simulink model "mechanical_characteristic_prsAD"  (R2015b)
settings: Solver=ode4  StartTime=0.0  StopTime=inf  FixedStep=2e-5  MaxStep=1e-6  RelTol=1e-6
libraries: powerlib x33, powerlib_meascontrol x4, simulink x1
settings Model: ExtModeTrigDuration=100  Creator=Alexey  LastModifiedBy=Артем
settings SolverCC: MaxConsecutiveZCs=1000000  ZeroCrossControl=DisableAll
settings DataIOCC: Decimation=10  LimitDataPoints=off  SaveFinalState=on  SaveFormat=StructureWithTime  SignalLoggingSaveFormat=ModelDataLogs  SaveOutput=off  SaveState=on  StateSaveName=tmp_raccel_xout  SignalLoggingName=tmp_raccel_logsout
settings OptimizationCC: ExpressionDepthLimit=2147483647  InitFltsAndDblsToZero=on  EfficientMapNaN2IntZero=off
settings DebuggingCC: SaveWithParameterizedLinksMsg=none  UnderspecifiedInitializationDetection=Classic  MergeDetectMultiDrivingBlocksExec=none  SignalResolutionControl=TryResolveAllWithWarning  SolverPrmCheckMsg=warning  MultiTaskDSMMsg=warning  MultiTaskCondExecSysMsg=none  FcnCallInpInsideContextMsg=UseLocalSettings  UnconnectedInputMsg=none  UnconnectedOutputMsg=none  UnconnectedLineMsg=none  StateNameClashWarn=warning
settings HardwareCC: ProdBitPerPointer=32  ProdLargestAtomicFloat=None  ProdIntDivRoundTo=Undefined  ProdEndianess=Unspecified  ProdWordSize=32  ProdHWDeviceType=32-bit Generic  TargetBitPerPointer=64  TargetLongLongMode=on  TargetIntDivRoundTo=Zero  TargetEndianess=LittleEndian  TargetWordSize=64  TargetHWDeviceType=MATLAB Host  ProdEqTarget=off
settings RTWCC: SystemTargetFile=raccel.tlc  TemplateMakefile=raccel_default_tmf  RTWVerbose=off  RTWUseSimCustomCode=on
settings CodeAppCC: GenerateComments=off  MaxIdLength=128  MangleLength=10  SimulinkBlockComments=off
settings RaccelTargetCC: ERTMultiwordTypeDef=System defined  ERTMultiwordLength=256  GeneratePreprocessorConditionals=Use local settings  ERTFirstTimeCompliant=off  MultiInstanceERTCode=off  ENABLE_SLEXEC_SSBRIDGE=0  RTWCAPIParams=on
settings ConfigComp: CovModelRefEnable=Off

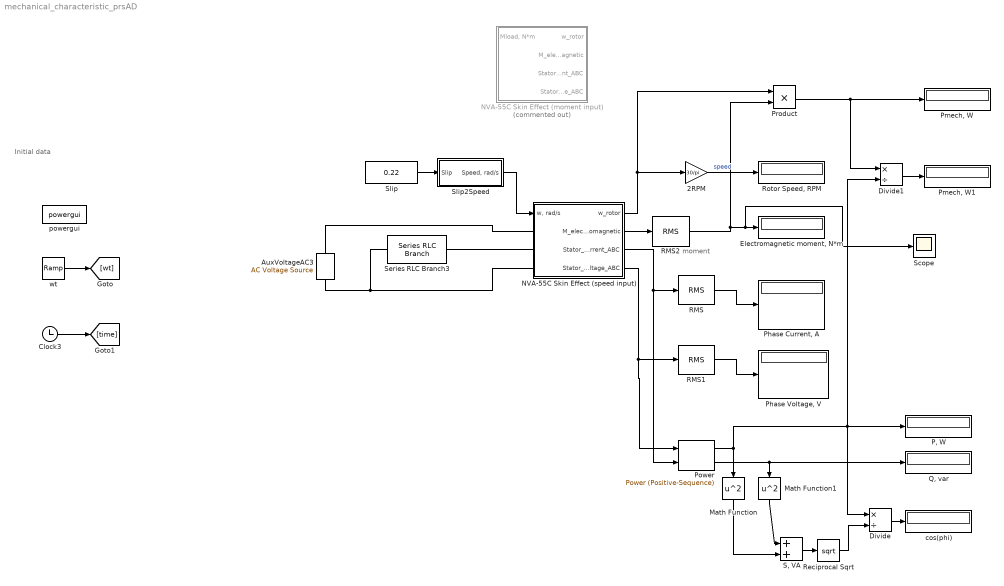
== system mechanical_characteristic_prsAD ==
  note: Initial data
  note: moment
  2RPM : Gain  Gain=30/pi
  AuxVoltageAC3 : powerlib/Electrical Sources/AC Voltage Source  Amplitude=278*sqrt(2)  Phase=0  Frequency=50  SampleTime=0  Measurements=None  BusType=swing  Pref=10e3  Qref=0  Qmin=-inf  Qmax=+inf
  Clock3 : Clock
  Divide : Product  Inputs=*/
  Divide1 : Product  Inputs=*/
  "Electromagnetic moment, N*m" : Display
  Math Function : Math  Operator=square  SaturateOnIntegerOverflow=on
  Math Function1 : Math  Operator=square  SaturateOnIntegerOverflow=on
  NVA-55C Skin Effect (moment input) : Subsystem  RequirementInfo={} %GIDa_83907570_a8f5_4683_9026_05a41bdf487c  Commented=on  mask(Модель асинхронной машины){f_nominal=50, Rs=0.0472, ls=0.0003883, Rr=0.0392, lr=0.0005399, Lm=0.011, Zp=2, Jr=1.25, l_s=326, q_s=119.52, n_2=38, d_r=207.4, q_r=498.1, h_p=3}
      mask prompts: f_nominal "Номинальная частота, Гц"; Rs "Активное сопротивление статора, Ом"; ls "Индуктивность статора, Гн"; Rr "Активное сопротивление ротора, Ом"; lr "Индуктивность ротора, Гн"; Lm "Взаимная индуктивность, Гн"; Zp "Число пар полюсов"; Jr "Коэффициент инерции ротора, кг*м^2"; l_s "Длина стержня ротора, мм"; q_s "Площадь поперечного сечения стержня, мм^2"; n_2 "Число пазов ротора"; d_r "Средний диаметр кольца, мм"; q_r "Площадь поперечного сечения кольца, мм^2"; h_p "Глубина паза, см"
      mask help: Описание
      mask init:
      | Ls = ls + Lm;
      | Lr = lr + Lm;
      | Kr = Lm / Lr;
      | Ks = Lm / Ls;
      | sigma = 1 - (Lm ^ 2) / (Ls * Lr);
      | 
      | dol_paz = (l_s / q_s) / ((l_s / q_s) + (n_2 * d_r) / (q_r * 2 * pi * Zp ^ 2));
      | dol_lob = ((n_2 * d_r) / (q_r * 2 * pi * Zp ^ 2))/ ((l_s / q_s) + (n_2 * d_r) / (q_r * 2 * pi * Zp ^ 2));
      | 
      | w_s = (2 * pi * f_nominal) / Zp;
  NVA-55C Skin Effect (speed input) : Subsystem  RequirementInfo={} %GIDa_29323b18_8ff0_47b3_9951_5813d07141ee  mask(Модель асинхронной машины){f_nominal=50, Rs=0.0472, ls=0.0003883, Rr=0.0392, lr=0.0005399, Lm=0.011, Zp=2, Jr=1.25, l_s=326, q_s=119.52, n_2=38, d_r=207.4, q_r=498.1, h_p=3}
      mask prompts: f_nominal "Номинальная частота, Гц"; Rs "Активное сопротивление статора, Ом"; ls "Индуктивность статора, Гн"; Rr "Активное сопротивление ротора, Ом"; lr "Индуктивность ротора, Гн"; Lm "Взаимная индуктивность, Гн"; Zp "Число пар полюсов"; Jr "Коэффициент инерции ротора, кг*м^2"; l_s "Длина стержня ротора, мм"; q_s "Площадь поперечного сечения стержня, мм^2"; n_2 "Число пазов ротора"; d_r "Средний диаметр кольца, мм"; q_r "Площадь поперечного сечения кольца, мм^2"; h_p "Глубина паза, см"
      mask help: Описание
      mask init: same as mechanical_characteristic_prsAD/NVA-55C Skin Effect (moment input)
  "P, W" : Display
  "Phase Current, A" : Display
  "Phase Voltage, V" : Display
  "Pmech, W" : Display
  "Pmech, W1" : Display
  Power : powerlib_meascontrol/Measurements/Power (Positive-Sequence)  Freq=50  Vinit=[0, 0]  Iinit=[0, 0]  Ts=0
  Product : Product
  "Q, var" : Display
  RMS : powerlib_meascontrol/Measurements/RMS  TrueRMS=on  Freq=50  RMSInit=0  Ts=0
  RMS1 : powerlib_meascontrol/Measurements/RMS  TrueRMS=on  Freq=50  RMSInit=0  Ts=0
  RMS2 : powerlib_meascontrol/Measurements/RMS  TrueRMS=on  Freq=50  RMSInit=0  Ts=0
  Reciprocal Sqrt : Sqrt  SaturateOnIntegerOverflow=on
  "Rotor Speed, RPM" : Display
  "S, VA" : Sum
  Scope : Scope
  Series RLC Branch3 : powerlib/Elements/Series RLC Branch  LConnTagsString=__new0  RConnTagsString=__new0  BranchType=C  Resistance=0  Inductance=0  SetiL0=off  InitialCurrent=0  Capacitance=2160e-6  Setx0=off  InitialVoltage=0  Measurements=None
  Slip : Constant  Value=0.22
  Slip2Speed : Subsystem  mask(Slip2Speed){w1=1500}
      mask prompts: w1 "Синхронная частота вращения, об/мин"
  cos(phi) : Display
  powergui : powerlib/powergui  SimulationMode=Discrete  SolverType=Tustin  SampleTime=2e-5  frequency=50  SPID=off  DisableSnubberDevices=off  DisableRonSwitches=off  DisableVfSwitches=off  SwTol=0  DisplayEquations=off  Interpol=off  ExternalGateDelay=off  methode=off  Ts=0  FunctionMessages=off  echomessages=off  HookPort=off  EnableUseOfTLC=off  x0status=blocks  frequencyindice=50  Pbase=100e6  ErrMax=1e-4  Iterations=50  UnitsV=kV  UnitsW=MW  buscounter=0  RestoreLinks=warning  ResistiveCurrentMeasurement=off  Frange=[0:2:500]  Ylog=off  Xlog=on  ShowGrid=off  save=off  variable=ZData  structure=0  ZoomFFT=on  StartTime=0.0  cycles=1  DisplayStyle=1  fundamental=60  FreqAxis=off  MaxFrequency=1000  frequencyindicesteady=1  RmsSteady=1  display=off
  wt : simulink/Sources/Ramp  slope=2*pi*50  start=0  X0=0
  wires:
  wt/1 -> [wt]
  Clock3/1 -> [time]
  2RPM/1 -> "Rotor Speed, RPM"/1  "speed"
  Slip/1 -> Slip2Speed/1(Slip)
  Slip2Speed/1("Speed, rad/s") -> NVA-55C Skin Effect (speed input)/1("w, rad/s")
  NVA-55C Skin Effect (speed input)/2(M_electromagnetic) -> RMS2/1
  NVA-55C Skin Effect (speed input)/1(w_rotor) -> 2RPM/1, Product/1
  NVA-55C Skin Effect (speed input)/3(Stator_current_ABC) -> RMS/1, Power/2
  NVA-55C Skin Effect (speed input)/4(Stator_voltage_ABC) -> Power/1, RMS1/1
  RMS/1 -> "Phase Current, A"/1
  RMS1/1 -> "Phase Voltage, V"/1
  Power/1 -> Divide/1, "P, W"/1, Divide1/2, Math Function/1
  Power/2 -> "Q, var"/1, Math Function1/1
  "S, VA"/1 -> Reciprocal Sqrt/1
  Divide/1 -> cos(phi)/1
  Product/1 -> Divide1/1, "Pmech, W"/1
  Divide1/1 -> "Pmech, W1"/1
  Math Function/1 -> "S, VA"/2
  Math Function1/1 -> "S, VA"/1
  Reciprocal Sqrt/1 -> Divide/2
  RMS2/1 -> Product/2, Scope/1, "Electromagnetic moment, N*m"/1
  connections:
  Series RLC Branch3/RConn1 -- NVA-55C Skin Effect (speed input)/LConn2
  AuxVoltageAC3/LConn1 -- NVA-55C Skin Effect (speed input)/LConn3 -- Series RLC Branch3/LConn1
  AuxVoltageAC3/RConn1 -- NVA-55C Skin Effect (speed input)/LConn1

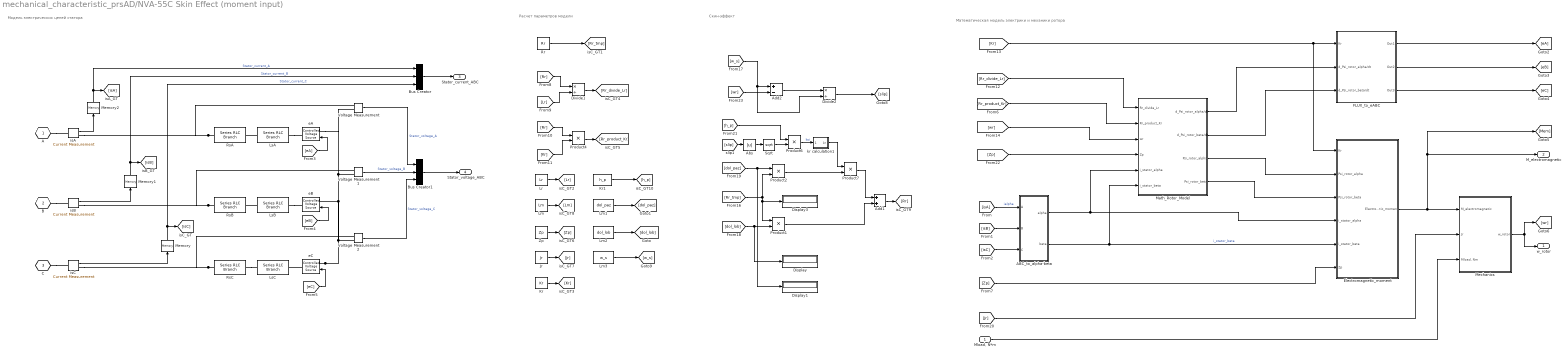
== system mechanical_characteristic_prsAD/NVA-55C Skin Effect (moment input) ==
  note: Модель электрических цепей статора
  note: Расчет параметров модели
  note: Математическая модель электрики и механики ротора
  note: Скин-эффект
  "Mload, N*m " : Inport
  ABC_to_alpha-beta : Subsystem
  Abs : Abs
  Add1 : Sum
  Add2 : Sum  Inputs=+-
  Bus Creator : BusCreator  Inputs=3
  Bus Creator1 : BusCreator  Inputs=3
  Display : Display
  Display1 : Display
  Display3 : Display
  Divide1 : Product  Inputs=*/
  Divide2 : Product  Inputs=*/
  "Electromagnetic_moment " : Subsystem
  FLUX_to_eABC : Subsystem
  Jr : Constant  Value=Jr
  Kr : Constant  Value=Kr
  Kr1 : Constant  Value=h_p
  Lm : Constant  Value=Lm
  Lm1 : Constant  Value=dol_paz
  Lm2 : Constant  Value=dol_lob
  Lm3 : Constant  Value=w_s
  Lr : Constant  Value=Lr
  LsA : powerlib/Elements/Series RLC Branch  LConnTagsString=__new0  RConnTagsString=__new0  BranchType=L  Resistance=Rs  Inductance=Ls * sigma  SetiL0=off  InitialCurrent=0  Capacitance=1e-6  Setx0=off  InitialVoltage=0  Measurements=None
  LsB : powerlib/Elements/Series RLC Branch  LConnTagsString=__new0  RConnTagsString=__new0  BranchType=L  Resistance=Rs  Inductance=Ls * sigma  SetiL0=off  InitialCurrent=0  Capacitance=1e-6  Setx0=off  InitialVoltage=0  Measurements=None
  LsC : powerlib/Elements/Series RLC Branch  LConnTagsString=__new0  RConnTagsString=__new0  BranchType=L  Resistance=Rs  Inductance=Ls * sigma  SetiL0=off  InitialCurrent=0  Capacitance=1e-6  Setx0=off  InitialVoltage=0  Measurements=None
  Math_Rotor_Model : Subsystem
  Mechanics : Subsystem
  Memory : Memory
  Memory1 : Memory
  Memory2 : Memory
  Product{1..2,4,6..7} (5 alike) : Product
  Rr : Constant  Value=Rr
  RsA : powerlib/Elements/Series RLC Branch  LConnTagsString=__new0  RConnTagsString=__new0  BranchType=R  Resistance=Rs  Inductance=1e-3  SetiL0=off  InitialCurrent=0  Capacitance=1e-6  Setx0=off  InitialVoltage=0  Measurements=None
  RsB : powerlib/Elements/Series RLC Branch  LConnTagsString=__new0  RConnTagsString=__new0  BranchType=R  Resistance=Rs  Inductance=1e-3  SetiL0=off  InitialCurrent=0  Capacitance=1e-6  Setx0=off  InitialVoltage=0  Measurements=None
  RsC : powerlib/Elements/Series RLC Branch  LConnTagsString=__new0  RConnTagsString=__new0  BranchType=R  Resistance=Rs  Inductance=1e-3  SetiL0=off  InitialCurrent=0  Capacitance=1e-6  Setx0=off  InitialVoltage=0  Measurements=None
  Sqrt : Sqrt  SaturateOnIntegerOverflow=on
  Voltage Measurement : powerlib/Measurements/Voltage Measurement  PhasorSimulation=off  OutputType=Complex  PSBequivalent=0
  Voltage Measurement1 : powerlib/Measurements/Voltage Measurement  PhasorSimulation=off  OutputType=Complex  PSBequivalent=0
  Voltage Measurement2 : powerlib/Measurements/Voltage Measurement  PhasorSimulation=off  OutputType=Complex  PSBequivalent=0
  Zp : Constant  Value=Zp
  eA : powerlib/Electrical Sources/Controlled Voltage Source  Initialize=on  Source_Type=AC  Amplitude=0  Phase=0  Frequency=0  Measurements=None
  eB : powerlib/Electrical Sources/Controlled Voltage Source  Initialize=on  Source_Type=AC  Amplitude=0  Phase=0  Frequency=0  Measurements=None
  eC : powerlib/Electrical Sources/Controlled Voltage Source  Initialize=on  Source_Type=AC  Amplitude=0  Phase=0  Frequency=0  Measurements=None
  isA : powerlib/Measurements/Current Measurement  PhasorSimulation=off  OutputType=Complex  PSBequivalent=0
  isB : powerlib/Measurements/Current Measurement  PhasorSimulation=off  OutputType=Complex  PSBequivalent=0
  isC : powerlib/Measurements/Current Measurement  PhasorSimulation=off  OutputType=Complex  PSBequivalent=0
  kr calculation1 : Subsystem
  A : PMIOPort  Tag=PMCPort  Port=1  Side=Left
  B : PMIOPort  Tag=PMCPort  Port=2  Side=Left
  C : PMIOPort  Tag=PMCPort  Port=3  Side=Left
  w_rotor : Outport
  M_electromagnetic : Outport  Port=2
  Stator_current_ABC : Outport  Port=3
  Stator_voltage_ABC : Outport  Port=4
  wires:
  kr calculation1/1(kr) -> Product7/1
  Bus Creator1/1 -> Stator_voltage_ABC/1
  Voltage Measurement2/1 -> Bus Creator1/3  "Stator_voltage_C"
  Voltage Measurement1/1 -> Bus Creator1/2  "Stator_voltage_B"
  Voltage Measurement/1 -> Bus Creator1/1  "Stator_voltage_A"
  Abs/1 -> Sqrt/1
  [slip] -> Abs/1
  [Jr] -> Mechanics/2(Jr)
  Divide2/1 -> [slip]
  Add2/1 -> Divide2/1
  [wr] -> Add2/2
  [w_s] -> Divide2/2, Add2/1
  Lm3/1 -> [w_s]
  Lm1/1 -> [dol_paz]
  Lm2/1 -> [dol_lob]
  Product7/1 -> Add1/1
  Product6/1 -> kr calculation1/1(ksi)  "ksi"
  Product2/1 -> Product7/2
  [h_p] -> Product6/1
  Sqrt/1 -> Product6/2
  Kr1/1 -> [h_p]
  Add1/1 -> [Rr]
  Product1/1 -> Add1/2
  [dol_paz] -> Product2/1, Display1/1
  [dol_lob] -> Product1/2, Display/1
  [Rr_tmp] -> Product2/2, Product1/1, Display3/1
  Rr/1 -> [Rr_tmp]
  [Zp] -> Math_Rotor_Model/4(Zp)
  [wr] -> Math_Rotor_Model/3(wr)
  [Zp] -> "Electromagnetic_moment "/6(Zp)
  Math_Rotor_Model/3(Psi_rotor_alpha) -> "Electromagnetic_moment "/2(Psi_rotor_alpha)
  Math_Rotor_Model/4(Psi_rotor_beta) -> "Electromagnetic_moment "/3(Psi_rotor_beta)
  Math_Rotor_Model/2(d_Psi_rotor_beta/dt) -> FLUX_to_eABC/3(d_Psi_rotor_beta/dt)
  Math_Rotor_Model/1(d_Psi_rotor_alpha/dt) -> FLUX_to_eABC/2(d_Psi_rotor_alpha/dt)
  [Rr_product_Kr] -> Math_Rotor_Model/2(Rr_product_Kr)
  [Rr_divide_Lr] -> Math_Rotor_Model/1(Rr_divide_Lr)
  FLUX_to_eABC/3(Out3) -> [eC]
  FLUX_to_eABC/2(Out2) -> [eB]
  FLUX_to_eABC/1(Out1) -> [eA]
  [Kr] -> FLUX_to_eABC/1(Kr), "Electromagnetic_moment "/1(Kr)
  "Electromagnetic_moment "/1(Electromagnetic_moment) -> [Mem], M_electromagnetic/1, Mechanics/1(M_electromagnetic)
  Bus Creator/1 -> Stator_current_ABC/1
  ABC_to_alpha-beta/1(alpha) -> "Electromagnetic_moment "/4(i_stator_alpha), Math_Rotor_Model/5(i_stator_alpha)
  [isC] -> ABC_to_alpha-beta/3(C)
  [isB] -> ABC_to_alpha-beta/2(B)
  ABC_to_alpha-beta/2(beta) -> "Electromagnetic_moment "/5(i_stator_beta), Math_Rotor_Model/6(i_stator_beta)  "i_stator_beta"
  Memory2/1 -> [isA], Bus Creator/1  "Stator_current_A"
  Memory1/1 -> [isB], Bus Creator/2  "Stator_current_B"
  Memory/1 -> [isC], Bus Creator/3  "Stator_current_C"
  isA/1 -> Memory2/1
  isB/1 -> Memory1/1
  isC/1 -> Memory/1
  Kr/1 -> [Kr]
  Lm/1 -> [Lm]
  [isA] -> ABC_to_alpha-beta/1(A)  "ialpha"
  Product4/1 -> [Rr_product_Kr]
  [Kr] -> Product4/2
  [Rr] -> Product4/1
  [eC] -> eC/1
  [eA] -> eA/1
  [eB] -> eB/1
  [Rr] -> Divide1/1
  Lr/1 -> [Lr]
  Jr/1 -> [Jr]
  Zp/1 -> [Zp]
  Divide1/1 -> [Rr_divide_Lr]
  [Lr] -> Divide1/2
  Mechanics/1(w_rotor) -> [wr], w_rotor/1
  "Mload, N*m "/1 -> Mechanics/3("Mload, Nm")
  connections:
  LsB/RConn1 -- eB/RConn1
  eC/LConn1 -- Voltage Measurement2/LConn2 -- eB/LConn1 -- Voltage Measurement1/LConn2 -- Voltage Measurement/LConn2 -- eA/LConn1
  LsA/RConn1 -- eA/RConn1
  eC/RConn1 -- LsC/RConn1
  RsA/LConn1 -- Voltage Measurement/LConn1 -- isA/RConn1
  A/RConn1 -- isA/LConn1
  RsB/LConn1 -- Voltage Measurement1/LConn1 -- isB/RConn1
  B/RConn1 -- isB/LConn1
  RsC/LConn1 -- Voltage Measurement2/LConn1 -- isC/RConn1
  C/RConn1 -- isC/LConn1
  LsA/LConn1 -- RsA/RConn1
  RsC/RConn1 -- LsC/LConn1
  LsB/LConn1 -- RsB/RConn1

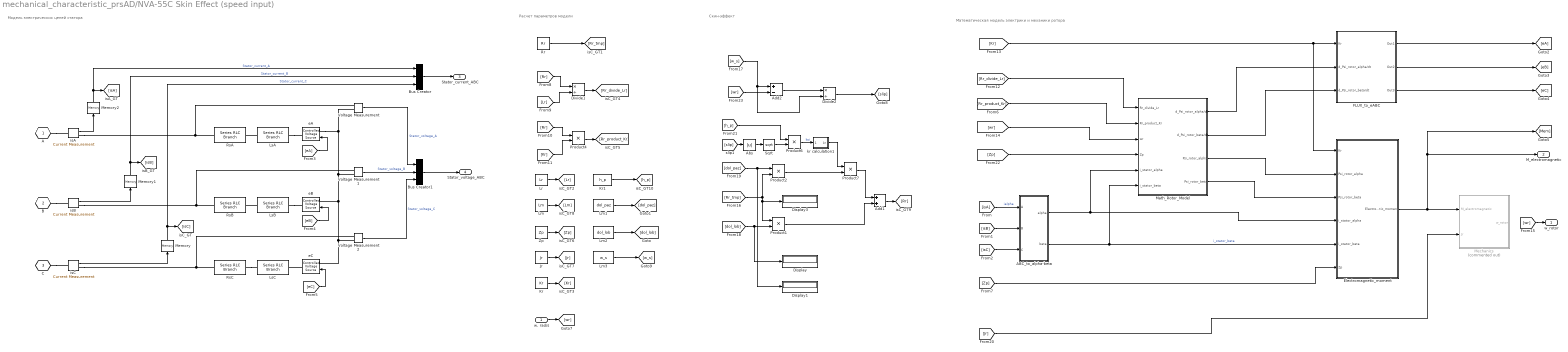
== system mechanical_characteristic_prsAD/NVA-55C Skin Effect (speed input) ==
  note: Скин-эффект
  note: Математическая модель электрики и механики ротора
  note: Расчет параметров модели
  note: Модель электрических цепей статора
  "w, rad/s" : Inport
  ABC_to_alpha-beta : Subsystem
  Abs : Abs
  Add1 : Sum
  Add2 : Sum  Inputs=+-
  Bus Creator : BusCreator  Inputs=3
  Bus Creator1 : BusCreator  Inputs=3
  Display : Display
  Display1 : Display
  Display3 : Display
  Divide1 : Product  Inputs=*/
  Divide2 : Product  Inputs=*/
  "Electromagnetic_moment " : Subsystem
  FLUX_to_eABC : Subsystem
  Jr : Constant  Value=Jr
  Kr : Constant  Value=Kr
  Kr1 : Constant  Value=h_p
  Lm : Constant  Value=Lm
  Lm1 : Constant  Value=dol_paz
  Lm2 : Constant  Value=dol_lob
  Lm3 : Constant  Value=w_s
  Lr : Constant  Value=Lr
  LsA : powerlib/Elements/Series RLC Branch  LConnTagsString=__new0  RConnTagsString=__new0  BranchType=L  Resistance=Rs  Inductance=Ls * sigma  SetiL0=off  InitialCurrent=0  Capacitance=1e-6  Setx0=off  InitialVoltage=0  Measurements=None
  LsB : powerlib/Elements/Series RLC Branch  LConnTagsString=__new0  RConnTagsString=__new0  BranchType=L  Resistance=Rs  Inductance=Ls * sigma  SetiL0=off  InitialCurrent=0  Capacitance=1e-6  Setx0=off  InitialVoltage=0  Measurements=None
  LsC : powerlib/Elements/Series RLC Branch  LConnTagsString=__new0  RConnTagsString=__new0  BranchType=L  Resistance=Rs  Inductance=Ls * sigma  SetiL0=off  InitialCurrent=0  Capacitance=1e-6  Setx0=off  InitialVoltage=0  Measurements=None
  Math_Rotor_Model : Subsystem
  Mechanics : Subsystem  Commented=on
  Memory : Memory
  Memory1 : Memory
  Memory2 : Memory
  Product{1..2,4,6..7} (5 alike) : Product
  Rr : Constant  Value=Rr
  RsA : powerlib/Elements/Series RLC Branch  LConnTagsString=__new0  RConnTagsString=__new0  BranchType=R  Resistance=Rs  Inductance=1e-3  SetiL0=off  InitialCurrent=0  Capacitance=1e-6  Setx0=off  InitialVoltage=0  Measurements=None
  RsB : powerlib/Elements/Series RLC Branch  LConnTagsString=__new0  RConnTagsString=__new0  BranchType=R  Resistance=Rs  Inductance=1e-3  SetiL0=off  InitialCurrent=0  Capacitance=1e-6  Setx0=off  InitialVoltage=0  Measurements=None
  RsC : powerlib/Elements/Series RLC Branch  LConnTagsString=__new0  RConnTagsString=__new0  BranchType=R  Resistance=Rs  Inductance=1e-3  SetiL0=off  InitialCurrent=0  Capacitance=1e-6  Setx0=off  InitialVoltage=0  Measurements=None
  Sqrt : Sqrt  SaturateOnIntegerOverflow=on
  Voltage Measurement : powerlib/Measurements/Voltage Measurement  PhasorSimulation=off  OutputType=Complex  PSBequivalent=0
  Voltage Measurement1 : powerlib/Measurements/Voltage Measurement  PhasorSimulation=off  OutputType=Complex  PSBequivalent=0
  Voltage Measurement2 : powerlib/Measurements/Voltage Measurement  PhasorSimulation=off  OutputType=Complex  PSBequivalent=0
  Zp : Constant  Value=Zp
  eA : powerlib/Electrical Sources/Controlled Voltage Source  Initialize=on  Source_Type=AC  Amplitude=0  Phase=0  Frequency=0  Measurements=None
  eB : powerlib/Electrical Sources/Controlled Voltage Source  Initialize=on  Source_Type=AC  Amplitude=0  Phase=0  Frequency=0  Measurements=None
  eC : powerlib/Electrical Sources/Controlled Voltage Source  Initialize=on  Source_Type=AC  Amplitude=0  Phase=0  Frequency=0  Measurements=None
  isA : powerlib/Measurements/Current Measurement  PhasorSimulation=off  OutputType=Complex  PSBequivalent=0
  isB : powerlib/Measurements/Current Measurement  PhasorSimulation=off  OutputType=Complex  PSBequivalent=0
  isC : powerlib/Measurements/Current Measurement  PhasorSimulation=off  OutputType=Complex  PSBequivalent=0
  kr calculation1 : Subsystem
  A : PMIOPort  Tag=PMCPort  Port=1  Side=Left
  B : PMIOPort  Tag=PMCPort  Port=2  Side=Left
  C : PMIOPort  Tag=PMCPort  Port=3  Side=Left
  w_rotor : Outport
  M_electromagnetic : Outport  Port=2
  Stator_current_ABC : Outport  Port=3
  Stator_voltage_ABC : Outport  Port=4
  wires:
  [wr] -> w_rotor/1
  "w, rad/s"/1 -> [wr]
  [Lr] -> Divide1/2
  Divide1/1 -> [Rr_divide_Lr]
  Zp/1 -> [Zp]
  Jr/1 -> [Jr]
  Lr/1 -> [Lr]
  [Rr] -> Divide1/1
  [eB] -> eB/1
  [eA] -> eA/1
  [eC] -> eC/1
  [Rr] -> Product4/1
  [Kr] -> Product4/2
  Product4/1 -> [Rr_product_Kr]
  [isA] -> ABC_to_alpha-beta/1(A)  "ialpha"
  Lm/1 -> [Lm]
  Kr/1 -> [Kr]
  isC/1 -> Memory/1
  isB/1 -> Memory1/1
  isA/1 -> Memory2/1
  Memory/1 -> Bus Creator/3, [isC]  "Stator_current_C"
  Memory1/1 -> Bus Creator/2, [isB]  "Stator_current_B"
  Memory2/1 -> Bus Creator/1, [isA]  "Stator_current_A"
  ABC_to_alpha-beta/2(beta) -> Math_Rotor_Model/6(i_stator_beta), "Electromagnetic_moment "/5(i_stator_beta)  "i_stator_beta"
  [isB] -> ABC_to_alpha-beta/2(B)
  [isC] -> ABC_to_alpha-beta/3(C)
  ABC_to_alpha-beta/1(alpha) -> Math_Rotor_Model/5(i_stator_alpha), "Electromagnetic_moment "/4(i_stator_alpha)
  Bus Creator/1 -> Stator_current_ABC/1
  "Electromagnetic_moment "/1(Electromagnetic_moment) -> Mechanics/1(M_electromagnetic), M_electromagnetic/1, [Mem]
  [Kr] -> "Electromagnetic_moment "/1(Kr), FLUX_to_eABC/1(Kr)
  FLUX_to_eABC/1(Out1) -> [eA]
  FLUX_to_eABC/2(Out2) -> [eB]
  FLUX_to_eABC/3(Out3) -> [eC]
  [Rr_divide_Lr] -> Math_Rotor_Model/1(Rr_divide_Lr)
  [Rr_product_Kr] -> Math_Rotor_Model/2(Rr_product_Kr)
  Math_Rotor_Model/1(d_Psi_rotor_alpha/dt) -> FLUX_to_eABC/2(d_Psi_rotor_alpha/dt)
  Math_Rotor_Model/2(d_Psi_rotor_beta/dt) -> FLUX_to_eABC/3(d_Psi_rotor_beta/dt)
  Math_Rotor_Model/4(Psi_rotor_beta) -> "Electromagnetic_moment "/3(Psi_rotor_beta)
  Math_Rotor_Model/3(Psi_rotor_alpha) -> "Electromagnetic_moment "/2(Psi_rotor_alpha)
  [Zp] -> "Electromagnetic_moment "/6(Zp)
  [wr] -> Math_Rotor_Model/3(wr)
  [Zp] -> Math_Rotor_Model/4(Zp)
  Rr/1 -> [Rr_tmp]
  [Rr_tmp] -> Display3/1, Product1/1, Product2/2
  [dol_lob] -> Display/1, Product1/2
  [dol_paz] -> Display1/1, Product2/1
  Product1/1 -> Add1/2
  Add1/1 -> [Rr]
  Kr1/1 -> [h_p]
  Sqrt/1 -> Product6/2
  [h_p] -> Product6/1
  Product2/1 -> Product7/2
  Product6/1 -> kr calculation1/1(ksi)  "ksi"
  Product7/1 -> Add1/1
  Lm2/1 -> [dol_lob]
  Lm1/1 -> [dol_paz]
  Lm3/1 -> [w_s]
  [w_s] -> Add2/1, Divide2/2
  [wr] -> Add2/2
  Add2/1 -> Divide2/1
  Divide2/1 -> [slip]
  [Jr] -> Mechanics/2(Jr)
  [slip] -> Abs/1
  Abs/1 -> Sqrt/1
  Voltage Measurement/1 -> Bus Creator1/1  "Stator_voltage_A"
  Voltage Measurement1/1 -> Bus Creator1/2  "Stator_voltage_B"
  Voltage Measurement2/1 -> Bus Creator1/3  "Stator_voltage_C"
  Bus Creator1/1 -> Stator_voltage_ABC/1
  kr calculation1/1(kr) -> Product7/1
  connections:
  LsB/LConn1 -- RsB/RConn1
  RsC/RConn1 -- LsC/LConn1
  LsA/LConn1 -- RsA/RConn1
  C/RConn1 -- isC/LConn1
  isC/RConn1 -- Voltage Measurement2/LConn1 -- RsC/LConn1
  B/RConn1 -- isB/LConn1
  isB/RConn1 -- Voltage Measurement1/LConn1 -- RsB/LConn1
  A/RConn1 -- isA/LConn1
  isA/RConn1 -- Voltage Measurement/LConn1 -- RsA/LConn1
  eC/RConn1 -- LsC/RConn1
  LsA/RConn1 -- eA/RConn1
  eA/LConn1 -- Voltage Measurement/LConn2 -- Voltage Measurement1/LConn2 -- eB/LConn1 -- Voltage Measurement2/LConn2 -- eC/LConn1
  LsB/RConn1 -- eB/RConn1

== system mechanical_characteristic_prsAD/Slip2Speed ==
  Slip : Inport
  Divide : Product  Inputs=**
  Subtract : Sum  Inputs=+-
  one1 : Constant
  one2 : Constant  Value=w1
  to rad/s : Gain  Gain=pi/30
  "Speed, rad/s" : Outport
  wires:
  Subtract/1 -> Divide/1
  one1/1 -> Subtract/1
  Divide/1 -> to rad/s/1
  to rad/s/1 -> "Speed, rad/s"/1
  Slip/1 -> Subtract/2
  one2/1 -> Divide/2

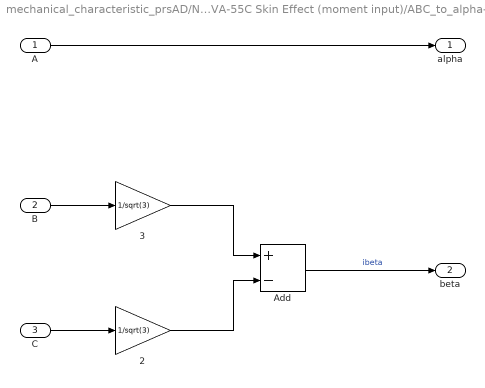
== system mechanical_characteristic_prsAD/NVA-55C Skin Effect (moment input)/ABC_to_alpha-beta ==
  A : Inport
  B : Inport  Port=2
  C : Inport  Port=3
  2 : Gain  Gain=1/sqrt(3)
  3 : Gain  Gain=1/sqrt(3)
  Add : Sum  Inputs=+-
  alpha : Outport
  beta : Outport  Port=2
  wires:
  A/1 -> alpha/1
  2/1 -> Add/2
  Add/1 -> beta/1  "ibeta"
  C/1 -> 2/1
  B/1 -> 3/1
  3/1 -> Add/1

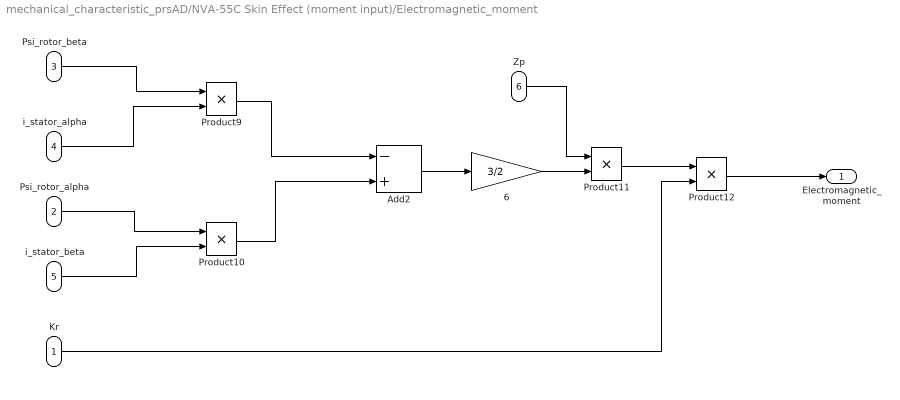
== system mechanical_characteristic_prsAD/NVA-55C Skin Effect (moment input)/Electromagnetic_moment  ==
  Kr : Inport
  Psi_rotor_alpha : Inport  Port=2
  Psi_rotor_beta : Inport  Port=3
  i_stator_alpha : Inport  Port=4
  i_stator_beta : Inport  Port=5
  Zp : Inport  Port=6
  6 : Gain  Gain=3/2
  Add2 : Sum  Inputs=-+
  Product{9..12} (4 alike) : Product
  Electromagnetic_moment : Outport
  wires:
  i_stator_beta/1 -> Product10/2
  Psi_rotor_beta/1 -> Product9/1
  Psi_rotor_alpha/1 -> Product10/1
  i_stator_alpha/1 -> Product9/2
  Add2/1 -> 6/1
  Zp/1 -> Product11/1
  6/1 -> Product11/2
  Product12/1 -> Electromagnetic_moment/1
  Product9/1 -> Add2/1
  Product10/1 -> Add2/2
  Kr/1 -> Product12/2
  Product11/1 -> Product12/1

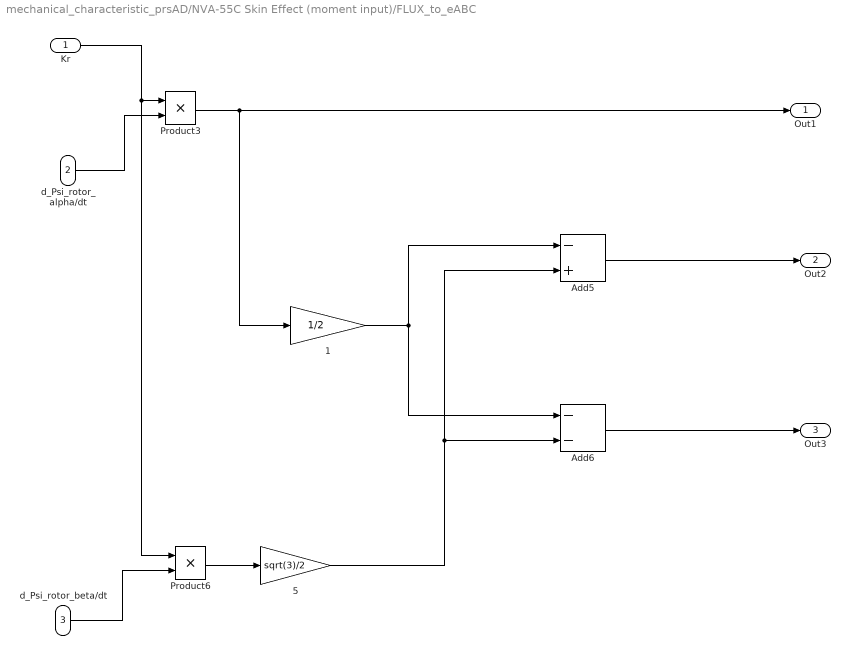
== system mechanical_characteristic_prsAD/NVA-55C Skin Effect (moment input)/FLUX_to_eABC ==
  Kr : Inport
  d_Psi_rotor_alpha/dt : Inport  Port=2
  d_Psi_rotor_beta/dt : Inport  Port=3
  1 : Gain  Gain=1/2
  5 : Gain  Gain=sqrt(3)/2
  Add5 : Sum  Inputs=-+
  Add6 : Sum  Inputs=--
  Product3 : Product
  Product6 : Product
  Out1 : Outport
  Out2 : Outport  Port=2
  Out3 : Outport  Port=3
  wires:
  d_Psi_rotor_beta/dt/1 -> Product6/2
  d_Psi_rotor_alpha/dt/1 -> Product3/2
  Add5/1 -> Out2/1
  Product3/1 -> 1/1, Out1/1
  Kr/1 -> Product3/1, Product6/1
  Add6/1 -> Out3/1
  5/1 -> Add6/2, Add5/2
  1/1 -> Add6/1, Add5/1
  Product6/1 -> 5/1

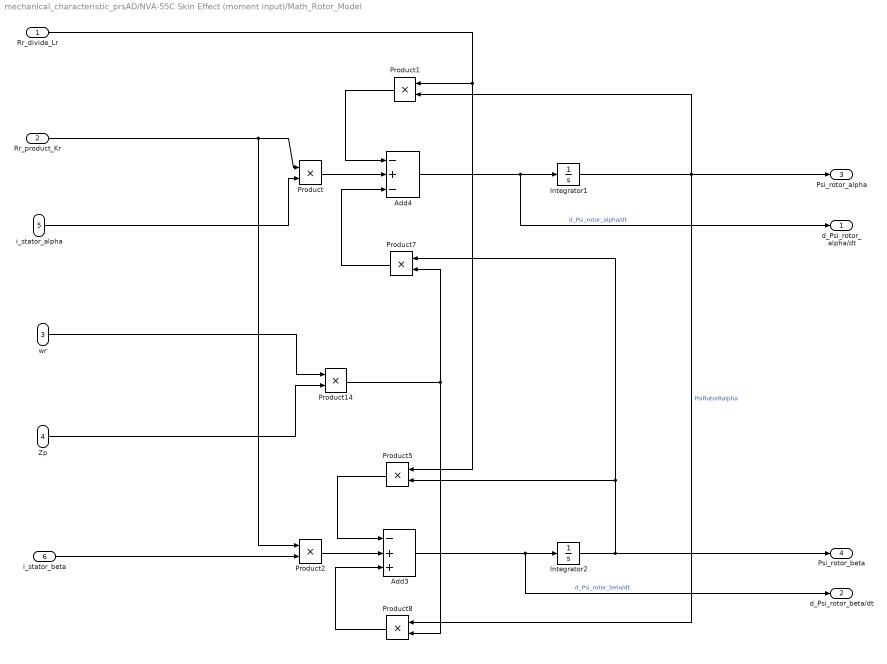
== system mechanical_characteristic_prsAD/NVA-55C Skin Effect (moment input)/Math_Rotor_Model ==
  Rr_divide_Lr : Inport
  Rr_product_Kr : Inport  Port=2
  wr : Inport  Port=3
  Zp : Inport  Port=4
  i_stator_alpha : Inport  Port=5
  i_stator_beta : Inport  Port=6
  Add3 : Sum  Inputs=-++
  Add4 : Sum  Inputs=-+-
  Integrator1 : Integrator
  Integrator2 : Integrator
  Product{,1..2,5,7..8,14} (7 alike) : Product
  d_Psi_rotor_alpha/dt : Outport
  d_Psi_rotor_beta/dt : Outport  Port=2
  Psi_rotor_alpha : Outport  Port=3
  Psi_rotor_beta : Outport  Port=4
  wires:
  i_stator_alpha/1 -> Product/2
  i_stator_beta/1 -> Product2/2
  Add4/1 -> Integrator1/1, d_Psi_rotor_alpha/dt/1  "d_Psi_rotor_alpha/dt"
  Integrator2/1 -> Psi_rotor_beta/1, Product7/1, Product5/2
  Add3/1 -> Integrator2/1, d_Psi_rotor_beta/dt/1  "d_Psi_rotor_beta/dt"
  Rr_divide_Lr/1 -> Product5/1, Product1/1
  Product8/1 -> Add3/3
  Product2/1 -> Add3/2
  Product/1 -> Add4/2
  wr/1 -> Product14/1
  Integrator1/1 -> Psi_rotor_alpha/1, Product8/1, Product1/2  "PsiRotorRalpha"
  Product5/1 -> Add3/1
  Rr_product_Kr/1 -> Product2/1, Product/1
  Product7/1 -> Add4/3
  Product1/1 -> Add4/1
  Product14/1 -> Product8/2, Product7/2
  Zp/1 -> Product14/2

== system mechanical_characteristic_prsAD/NVA-55C Skin Effect (moment input)/Mechanics ==
  M_electromagnetic : Inport
  Jr : Inport  Port=2
  "Mload, Nm" : Inport  Port=3
  Add1 : Sum  Inputs=+-
  Divide2 : Product  Inputs=*/
  Integrator3 : Integrator
  w_rotor : Outport
  wires:
  M_electromagnetic/1 -> Add1/1
  "Mload, Nm"/1 -> Add1/2
  Integrator3/1 -> Divide2/1
  Add1/1 -> Integrator3/1
  Jr/1 -> Divide2/2
  Divide2/1 -> w_rotor/1

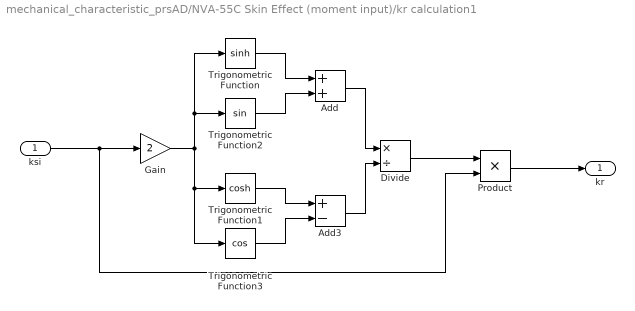
== system mechanical_characteristic_prsAD/NVA-55C Skin Effect (moment input)/kr calculation1 ==
  ksi : Inport
  Add : Sum
  Add3 : Sum  Inputs=+-
  Divide : Product  Inputs=*/
  Gain : Gain  Gain=2
  Product : Product
  Trigonometric Function : Trigonometry  Operator=sinh
  Trigonometric Function1 : Trigonometry  Operator=cosh
  Trigonometric Function2 : Trigonometry
  Trigonometric Function3 : Trigonometry  Operator=cos
  kr : Outport
  wires:
  Gain/1 -> Trigonometric Function/1, Trigonometric Function2/1, Trigonometric Function3/1, Trigonometric Function1/1
  Trigonometric Function2/1 -> Add/2
  Add/1 -> Divide/1
  Add3/1 -> Divide/2
  Product/1 -> kr/1
  Trigonometric Function/1 -> Add/1
  Divide/1 -> Product/1
  ksi/1 -> Product/2, Gain/1
  Trigonometric Function1/1 -> Add3/1
  Trigonometric Function3/1 -> Add3/2

== system mechanical_characteristic_prsAD/NVA-55C Skin Effect (speed input)/ABC_to_alpha-beta ==
  A : Inport
  B : Inport  Port=2
  C : Inport  Port=3
  2 : Gain  Gain=1/sqrt(3)
  3 : Gain  Gain=1/sqrt(3)
  Add : Sum  Inputs=+-
  alpha : Outport
  beta : Outport  Port=2
  wires:
  3/1 -> Add/1
  B/1 -> 3/1
  C/1 -> 2/1
  Add/1 -> beta/1  "ibeta"
  2/1 -> Add/2
  A/1 -> alpha/1

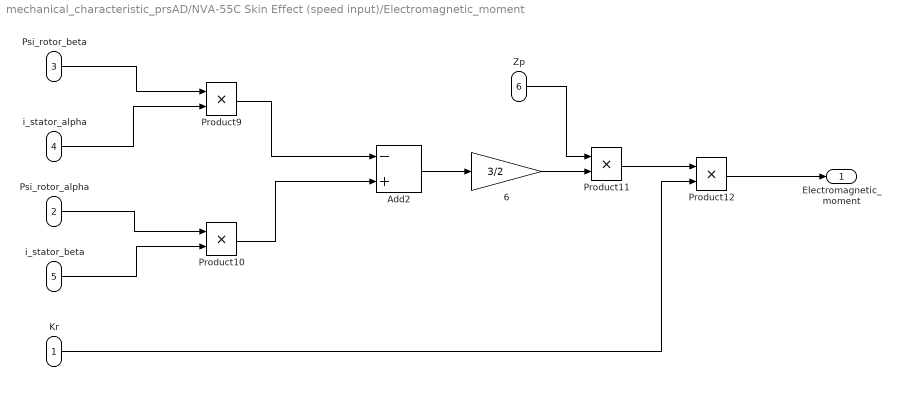
== system mechanical_characteristic_prsAD/NVA-55C Skin Effect (speed input)/Electromagnetic_moment  ==
  Kr : Inport
  Psi_rotor_alpha : Inport  Port=2
  Psi_rotor_beta : Inport  Port=3
  i_stator_alpha : Inport  Port=4
  i_stator_beta : Inport  Port=5
  Zp : Inport  Port=6
  6 : Gain  Gain=3/2
  Add2 : Sum  Inputs=-+
  Product{9..12} (4 alike) : Product
  Electromagnetic_moment : Outport
  wires:
  Product11/1 -> Product12/1
  Kr/1 -> Product12/2
  Product10/1 -> Add2/2
  Product9/1 -> Add2/1
  Product12/1 -> Electromagnetic_moment/1
  6/1 -> Product11/2
  Zp/1 -> Product11/1
  Add2/1 -> 6/1
  i_stator_alpha/1 -> Product9/2
  Psi_rotor_alpha/1 -> Product10/1
  Psi_rotor_beta/1 -> Product9/1
  i_stator_beta/1 -> Product10/2

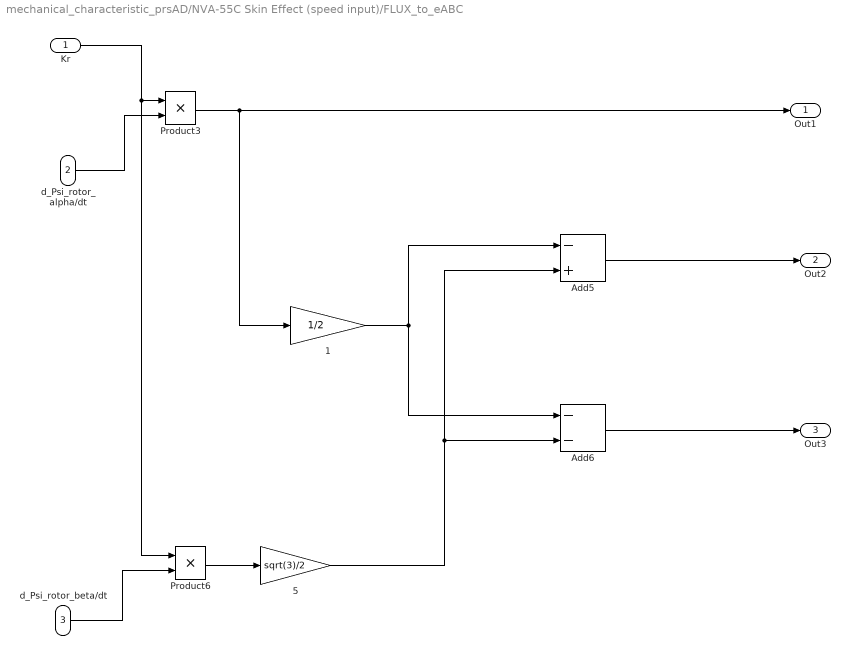
== system mechanical_characteristic_prsAD/NVA-55C Skin Effect (speed input)/FLUX_to_eABC ==
  Kr : Inport
  d_Psi_rotor_alpha/dt : Inport  Port=2
  d_Psi_rotor_beta/dt : Inport  Port=3
  1 : Gain  Gain=1/2
  5 : Gain  Gain=sqrt(3)/2
  Add5 : Sum  Inputs=-+
  Add6 : Sum  Inputs=--
  Product3 : Product
  Product6 : Product
  Out1 : Outport
  Out2 : Outport  Port=2
  Out3 : Outport  Port=3
  wires:
  Product6/1 -> 5/1
  1/1 -> Add5/1, Add6/1
  5/1 -> Add5/2, Add6/2
  Add6/1 -> Out3/1
  Kr/1 -> Product6/1, Product3/1
  Product3/1 -> Out1/1, 1/1
  Add5/1 -> Out2/1
  d_Psi_rotor_alpha/dt/1 -> Product3/2
  d_Psi_rotor_beta/dt/1 -> Product6/2

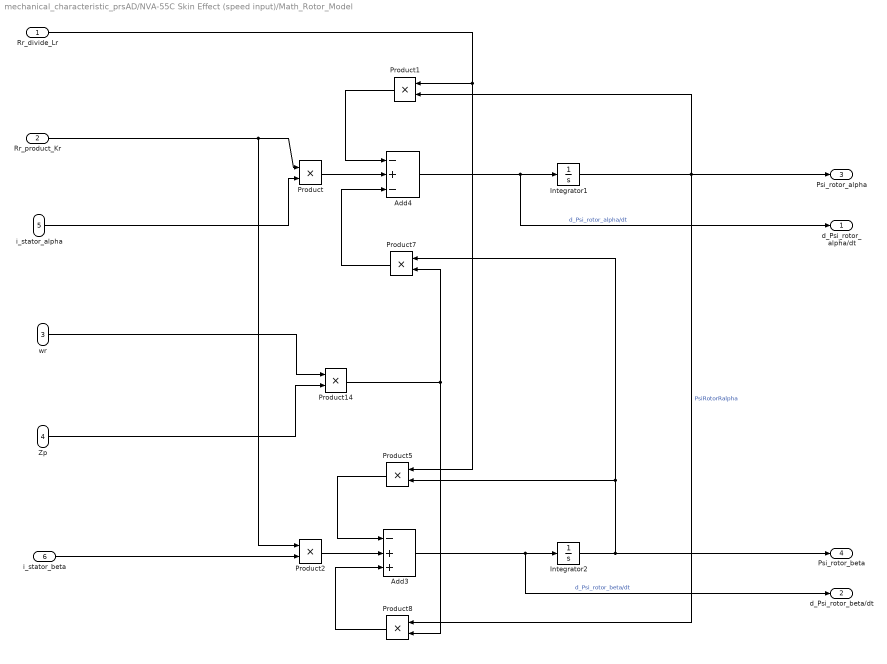
== system mechanical_characteristic_prsAD/NVA-55C Skin Effect (speed input)/Math_Rotor_Model ==
  Rr_divide_Lr : Inport
  Rr_product_Kr : Inport  Port=2
  wr : Inport  Port=3
  Zp : Inport  Port=4
  i_stator_alpha : Inport  Port=5
  i_stator_beta : Inport  Port=6
  Add3 : Sum  Inputs=-++
  Add4 : Sum  Inputs=-+-
  Integrator1 : Integrator
  Integrator2 : Integrator
  Product{,1..2,5,7..8,14} (7 alike) : Product
  d_Psi_rotor_alpha/dt : Outport
  d_Psi_rotor_beta/dt : Outport  Port=2
  Psi_rotor_alpha : Outport  Port=3
  Psi_rotor_beta : Outport  Port=4
  wires:
  Zp/1 -> Product14/2
  Product14/1 -> Product7/2, Product8/2
  Product1/1 -> Add4/1
  Product7/1 -> Add4/3
  Rr_product_Kr/1 -> Product/1, Product2/1
  Product5/1 -> Add3/1
  Integrator1/1 -> Product1/2, Product8/1, Psi_rotor_alpha/1  "PsiRotorRalpha"
  wr/1 -> Product14/1
  Product/1 -> Add4/2
  Product2/1 -> Add3/2
  Product8/1 -> Add3/3
  Rr_divide_Lr/1 -> Product1/1, Product5/1
  Add3/1 -> d_Psi_rotor_beta/dt/1, Integrator2/1  "d_Psi_rotor_beta/dt"
  Integrator2/1 -> Product5/2, Product7/1, Psi_rotor_beta/1
  Add4/1 -> d_Psi_rotor_alpha/dt/1, Integrator1/1  "d_Psi_rotor_alpha/dt"
  i_stator_beta/1 -> Product2/2
  i_stator_alpha/1 -> Product/2

== system mechanical_characteristic_prsAD/NVA-55C Skin Effect (speed input)/Mechanics ==
  M_electromagnetic : Inport
  Jr : Inport  Port=2
  Add1 : Sum  Inputs=+-
  Constant : Constant  Value=0
  Divide2 : Product  Inputs=*/
  Integrator3 : Integrator
  w_rotor : Outport
  wires:
  Divide2/1 -> w_rotor/1
  Jr/1 -> Divide2/2
  Add1/1 -> Integrator3/1
  Integrator3/1 -> Divide2/1
  Constant/1 -> Add1/2
  M_electromagnetic/1 -> Add1/1

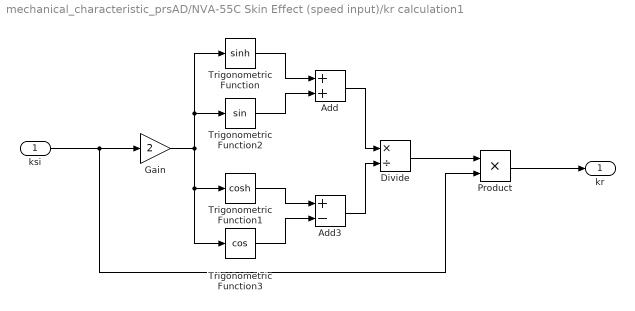
== system mechanical_characteristic_prsAD/NVA-55C Skin Effect (speed input)/kr calculation1 ==
  ksi : Inport
  Add : Sum
  Add3 : Sum  Inputs=+-
  Divide : Product  Inputs=*/
  Gain : Gain  Gain=2
  Product : Product
  Trigonometric Function : Trigonometry  Operator=sinh
  Trigonometric Function1 : Trigonometry  Operator=cosh
  Trigonometric Function2 : Trigonometry
  Trigonometric Function3 : Trigonometry  Operator=cos
  kr : Outport
  wires:
  Trigonometric Function3/1 -> Add3/2
  Trigonometric Function1/1 -> Add3/1
  ksi/1 -> Gain/1, Product/2
  Divide/1 -> Product/1
  Trigonometric Function/1 -> Add/1
  Product/1 -> kr/1
  Add3/1 -> Divide/2
  Add/1 -> Divide/1
  Trigonometric Function2/1 -> Add/2
  Gain/1 -> Trigonometric Function1/1, Trigonometric Function3/1, Trigonometric Function2/1, Trigonometric Function/1
